simulink model "velo"  (R2015a)
settings: Solver=ode3  StartTime=0.0  StopTime=20.0  FixedStep=ts  RelTol=1e-3
undefined symbols (not defined in the file): p_const, r_const, s_time, ts, u_ini
libraries: arduinolib x2
settings Model: SimulationMode=external  ExtModeTrigDuration=2  Creator=shohei  LastModifiedBy=shohei
settings DataIOCC: LimitDataPoints=off  SaveFormat=StructureWithTime  SaveOutput=off  SaveTime=off
settings OptimizationCC: OptimizeModelRefInitCode=on  LifeSpan=1
settings DebuggingCC: UnderspecifiedInitializationDetection=Classic  MergeDetectMultiDrivingBlocksExec=none
settings HardwareCC: ProdBitPerInt=16  ProdBitPerPointer=8  ProdIntDivRoundTo=Zero  ProdEndianess=LittleEndian  ProdWordSize=8  ProdHWDeviceType=Atmel->AVR
settings RTWCC: SystemTargetFile=realtime.tlc  GenerateMakefile=off  TemplateMakefile=realtime.tmf  Description=Run on Target Hardware  RTWVerbose=off
settings ERTTargetCC: CombineOutputUpdateFcns=off  ExtModeTransport=3  ExtModeMexFile=ext_serial_win32_comm_rtt  ExtModeMexArgs=0 1 9600  ERTSrcFileBannerTemplate=realtime_code_template.cgt  ERTHdrFileBannerTemplate=realtime_code_template.cgt  ERTDataSrcFileTemplate=realtime_code_template.cgt  ERTDataHdrFileTemplate=realtime_code_template.cgt  ERTCustomFileTemplate=realtime_file_process.tlc

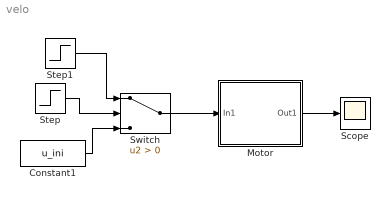
== system velo ==
  Constant1 : Constant  Value=u_ini
  "Motor " : Subsystem
  Scope : Scope
  Step : Step  SampleTime=ts
  Step1 : Step  Time=s_time  Before=r_const  After=p_const  SampleTime=ts
  Switch : Switch  Criteria=u2 > Threshold
  wires:
  Step/1 -> Switch/2
  Constant1/1 -> Switch/3
  Step1/1 -> Switch/1
  Switch/1 -> "Motor "/1(In1)
  "Motor "/1(Out1) -> Scope/1

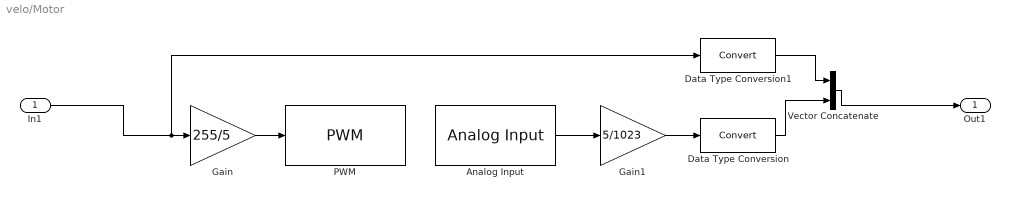
== system velo/Motor  ==
  In1 : Inport
  Analog Input : arduinolib/Analog Input  pinNumber=5  sampleTime=ts  blockPlatform=arduino
  Data Type Conversion : DataTypeConversion
  Data Type Conversion1 : DataTypeConversion
  Gain : Gain  Gain=255/5
  Gain1 : Gain  Gain=5/1023
  PWM : arduinolib/PWM  pinNumber=9  blockPlatform=arduino
  Vector Concatenate : Concatenate
  Out1 : Outport
  wires:
  Data Type Conversion/1 -> Vector Concatenate/2
  Gain1/1 -> Data Type Conversion/1
  Gain/1 -> PWM/1
  Analog Input/1 -> Gain1/1
  Data Type Conversion1/1 -> Vector Concatenate/1
  In1/1 -> Data Type Conversion1/1, Gain/1
  Vector Concatenate/1 -> Out1/1
